simulink model "Pendulum_Sim_Statespace_Poleplacement"  (R2023b)
settings: Solver=VariableStepAuto  StartTime=0.0  StopTime=20.0  RelTol=1e-3
values from neighbouring files (symbols this model uses):
  A = A_1\A_2    [Model_Adjusted.m]    (also in Model_Simplified.m; Phi.mat = [0.526224510393 -0.550606543846 1 0 0.00686239289147 -0.0307; Simulation_model_updated.m; Voltage.mat = [0.526224510393 -0.550606543846 1 0 0.00686239289147 -0.0307)
  B = A_1\B_1    [Model_Adjusted.m]    (also in Model_Simplified.m; Phi.mat = [12.5291550093 -13.1096796154 0 0]; Simulation_model_updated.m; Voltage.mat = [12.5291550093 -13.1096796154 0 0])
  C = eye(4)    [Model_Adjusted.m]    (also in Model_Simplified.m; Phi.mat = [1 0 0 0 0 1 0 0 0 0 1 0 ... (16 elements, 4x4)]; Simulation_model_updated.m = eye(5); Voltage.mat = [1 0 0 0 0 1 0 0 0 0 1 0 ... (16 elements, 4x4)])
  D = zeros(4,1)    [Model_Adjusted.m]    (also in Model_Simplified.m; Phi.mat = [0 0 0 0]; Simulation_model_updated.m = zeros(5,1); Voltage.mat = [0 0 0 0])
  K_pp = place(A,B,p1)    [Model_Adjusted.m]    (also in Model_Simplified.m; Phi.mat = [-1.23425797793 -4.23707061959 -1 -48.2020366551]; Simulation_model_updated.m = place(A,B,p); Voltage.mat = [-1.23425797793 -4.23707061959 -1 -48.2020366551])
settings Model: Creator=Asus  LastModifiedBy=Asus

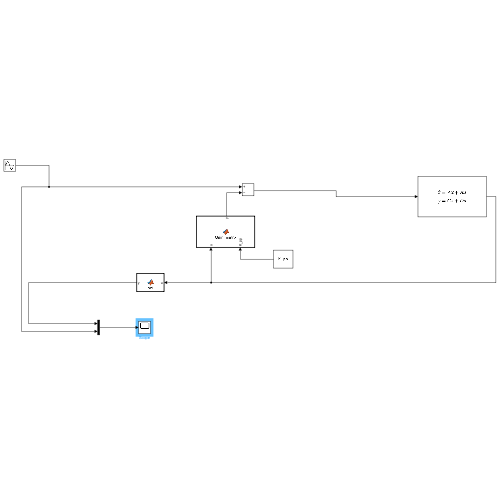
[thumbnail: Simulink's stored preview of the top-level diagram]
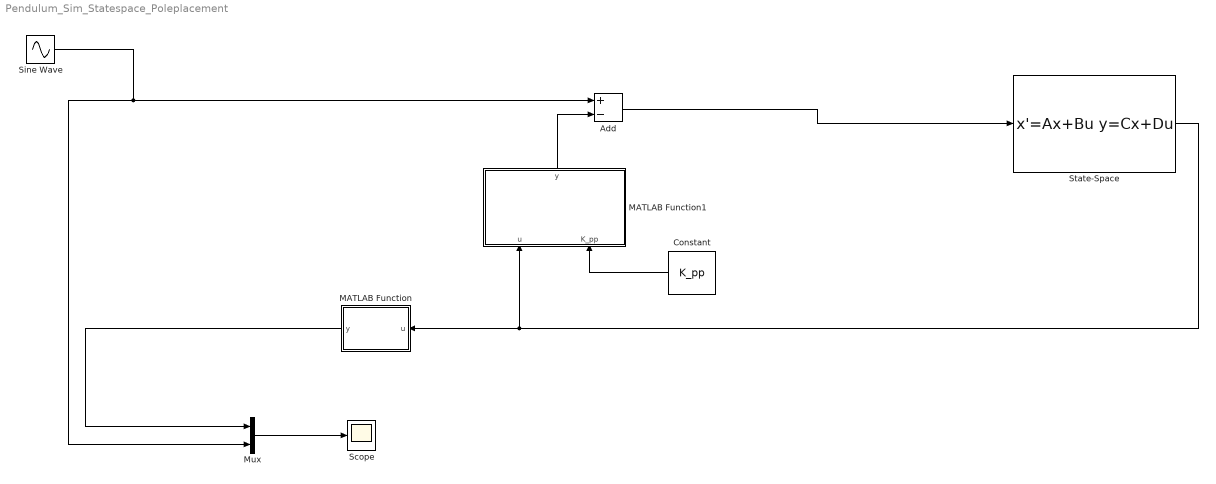
== system Pendulum_Sim_Statespace_Poleplacement ==
  Add : Sum  Inputs=+-
  Constant : Constant  Value=K_pp
  MATLAB Function : MATLAB Function  TreatAsAtomicUnit=on
  MATLAB Function1 : MATLAB Function  TreatAsAtomicUnit=on
  Mux : Mux  Inputs=2
  Scope : Scope
  Sine Wave : Sin  SampleTime=0
  State-Space : StateSpace  A=A  B=B  C=C  D=D  InitialCondition=0
  wires:
  Add/1 -> State-Space/1
  Sine Wave/1 -> Add/1, Mux/2
  Mux/1 -> Scope/1
  State-Space/1 -> MATLAB Function/1(u), MATLAB Function1/1(u)
  MATLAB Function/1(y) -> Mux/1
  MATLAB Function1/1(y) -> Add/2
  Constant/1 -> MATLAB Function1/2(K_pp)

== matlab function Pendulum_Sim_Statespace_Poleplacement/MATLAB Function ==
  data: u input; y output
function y = phi(u)

y = u(4);

end

== matlab function Pendulum_Sim_Statespace_Poleplacement/MATLAB Function1 ==
  data: u input; y output; K_pp input
function y = Gain_matrix(u, K_pp)
y = K_pp'*u;
end
